simulink model "cessnamodel"  (R2026a)
settings: Solver=VariableStepAuto
values from neighbouring files (symbols this model uses):
  u0 = [ ... (first row only)    [plot_flight_path.m]
  X0 = [ ... (first row only)    [plot_flight_path.m]
undefined symbols (not defined in the file or in its folder): cessna182_model
settings Model: Creator=nuris  LastModifiedBy=nuris

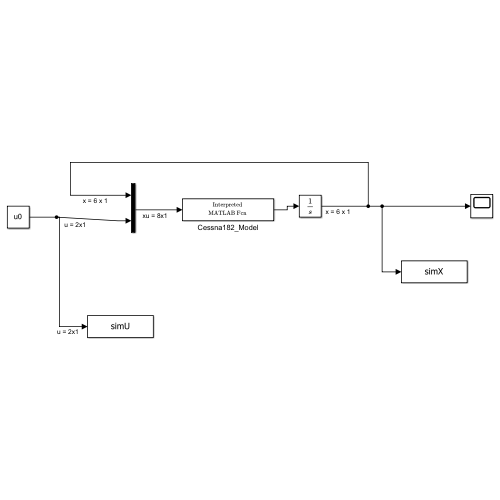
[thumbnail: Simulink's stored preview of the top-level diagram]
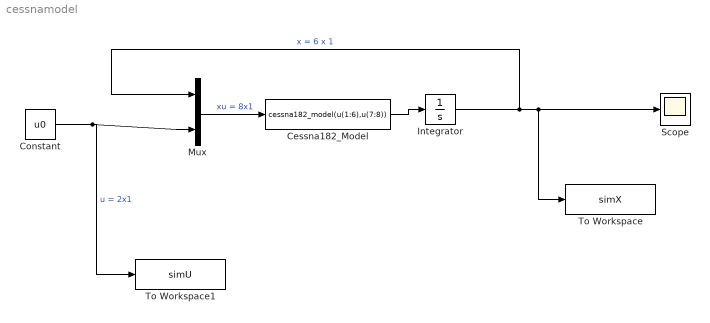
== system cessnamodel ==
  Cessna182_Model : MATLABFcn  MATLABFcn=cessna182_model(u(1:6),u(7:8))
  Constant : Constant  Value=u0
  Integrator : Integrator  InitialCondition=X0
  Mux : Mux  Inputs=2
  Scope : Scope
      settings: ActiveDisplayYMinimum=-2726.531512495636  ActiveDisplayYMaximum=775.87160354920707
  To Workspace : ToWorkspace  VariableName=simX  SaveFormat=Timeseries  SampleTime=-1
  To Workspace1 : ToWorkspace  VariableName=simU  SaveFormat=Timeseries  SampleTime=-1
  wires:
  Constant/1 -> To Workspace1/1, Mux/2  "u = 2x1"
  Cessna182_Model/1 -> Integrator/1
  Integrator/1 -> Mux/1, To Workspace/1, Scope/1  "x = 6 x 1"
  Mux/1 -> Cessna182_Model/1  "xu = 8x1"
